simulink model "VSI_fed_Induction_motor"  (R2021a)
settings: Solver=VariableStepAuto  StartTime=0.0  StopTime=10.0  RelTol=1e-3
undefined symbols (not defined in the file): Ts
libraries: spsStairGeneratorLib x3, spsVoltageMeasurementLib x3, spsThreePhaseSourceLib x1, spsMultimeterLib x1, electricdrivelib x1, spspowerguiLib x1
settings Model: Creator=suchi  LastModifiedBy=suchi

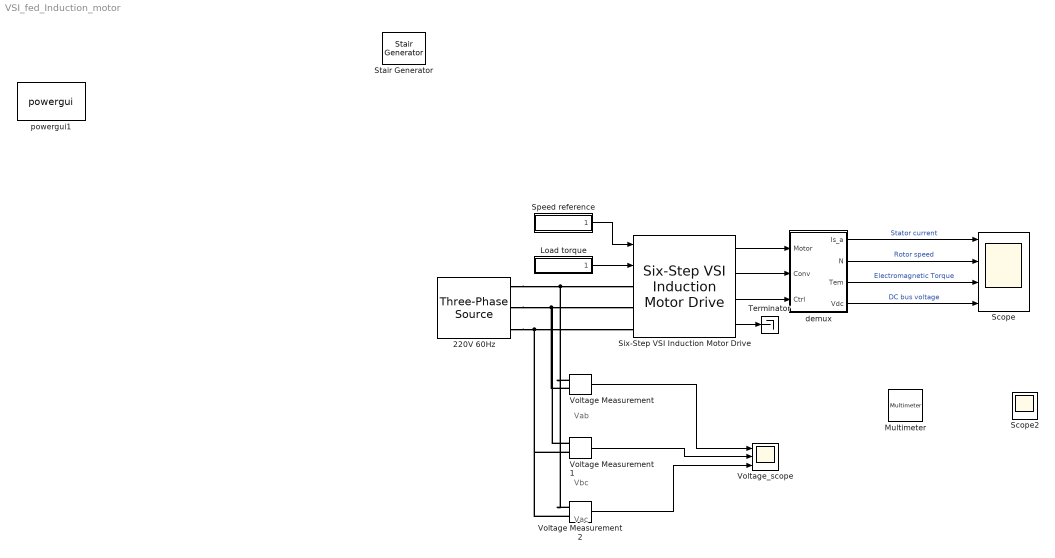
== system VSI_fed_Induction_motor ==
  note: Vac
  note: Vbc
  note: Vab
  220V 60Hz : spsThreePhaseSourceLib/Three-Phase Source  InternalConnection=Yg  VoltagePhases=off  Voltage=220  PhaseAngle=0  Voltage_phases=[25e3 25e3 25e3]/sqrt(3)  PhaseAngles_phases=[0 -120 +120]  Frequency=60  NonIdealSource=on  SpecifyImpedance=off  Resistance=0.1  Inductance=0.1e-3  ShortCircuitLevel=0  BaseVoltage=0  XRratio=0  BusType=swing  Pref=0  Qref=0  Prefabc=[10e3, 10e3, 10e3]  Qrefabc=[0, 0, 0]  Qmin=-inf  Qmax=inf
  Load torque : Subsystem
  Multimeter : spsMultimeterLib/Multimeter  PhasorSimulation=off  OutputType=Complex  sel=1  L=1  Gain=0  yselected={}  PSBOutputType=1  PSBequivalent=0  AxesSetting=[0,0.1,-100,100]  Display=0  SavedBlockNames=-11
  Scope : Scope  NumInputPorts=4
  Scope2 : Scope
  Six-Step VSI Induction Motor Drive : electricdrivelib/AC drives/Six-Step VSI Induction Motor Drive  ReferenceFrame=Stationary  IterativeDiscreteModel=Trapezoidal non iterative  Pn=2238  Vn=220  fn=60  Rs=0.435  Lls=0.002  Lms=69.31e-3  Rr=0.816  Llr=0.002  ia=0  pha=0  ib=0  phb=0  ic=0  phc=0  J=0.089  Friction=0.005  p=2  slip=1  thdeg=0  Rsnb_rec=5e3  Csnb_rec=100e-9  Ron_rec=1e-3  Vf_rec=1.3  ind_bus=1e-3  cap_bus=4000e-6  Rbrake=8  fbrake=4000  deviceType=IGBT / Diodes  Ron_inv=1e-3  Vf_inv=1.7  Vfd_inv=1.7  Tf=1e-6  Tt=2e-6  Tf_GTO=10e-6  Tt_GTO=20e-6  Rsnb_inv=1e3  Csnb_inv=20e-9  fc_busc=30  network_freq=60  bus_dev_neg=20  bus_dev_pos=20  kp_busc=0.01  ki_busc=0.1  busVolt_min=30  busVolt_max=280  Acc=2000  Dec=-2000  outfreq_min=0  outfreq_max=120  vh_ratio=5  zc_time=0.5  baseSampleTime=2e-05  outputBusMode=Multiple output buses  busLabels=off  MechanicalLoad=Torque Tm  driveType=AC1  AverageValue=off
      settings: SourceProductBaseCode=PS
  Speed reference : Subsystem
  Stair Generator : spsStairGeneratorLib/Stair Generator  t=[0, 1, 3, 3.5]  e=[1, -1, 2.5, 0]  Ts=0
  Terminator : Terminator
  Voltage Measurement : spsVoltageMeasurementLib/Voltage Measurement  PhasorSimulation=off  OutputType=Complex  PSBequivalent=0
  Voltage Measurement1 : spsVoltageMeasurementLib/Voltage Measurement  PhasorSimulation=off  OutputType=Complex  PSBequivalent=0
  Voltage Measurement2 : spsVoltageMeasurementLib/Voltage Measurement  PhasorSimulation=off  OutputType=Complex  PSBequivalent=0
  Voltage_scope : Scope  NumInputPorts=3
  demux : Subsystem
  powergui1 : spspowerguiLib/powergui  Priority=2  SimulationMode=Discrete  SampleTime=Ts  frequency=60  Iterations=50  frequencyindice=60  Pbase=100e6  ErrMax=1e-4  UnitsV=kV  UnitsW=MW  buscounter=0  FunctionMessages=off  echomessages=off  EnableUseOfTLC=off  CurrentSourceSwitches=off  DisableSnubberDevices=off  DisableRonSwitches=off  DisableVfSwitches=off  DisplayEquations=off  AutomaticDiscreteSolvers=off  SolverType=Tustin/Backward Euler (TBE)  Interpol=off  ExternalGateDelay=off  methode=off  Ts=0  x0status=blocks  SPID=off  SwTol=0  HookPort=off  NonlinearTolerance=1e-4  nMaxIteration=100  ContinueOnMaxIteration=off  RestoreLinks=warning  ResistiveCurrentMeasurement=off  Frange=[0:2:500]  Ylog=off  Xlog=on  ShowGrid=off  save=off  variable=ZData  structure=0  ZoomFFT=on  StartTime=0.0  cycles=1  DisplayStyle=1  fundamental=60  FreqAxis=off  MaxFrequency=1000  frequencyindicesteady=1  RmsSteady=1  display=off
  wires:
  Six-Step VSI Induction Motor Drive/2 -> demux/2(Conv)
  Load torque/1(" ") -> Six-Step VSI Induction Motor Drive/2
  demux/3(Tem) -> Scope/3  "Electromagnetic Torque"
  demux/4(Vdc) -> Scope/4  "DC bus voltage"
  Six-Step VSI Induction Motor Drive/4 -> Terminator/1
  demux/1(Is_a) -> Scope/1  "Stator current"
  Six-Step VSI Induction Motor Drive/3 -> demux/3(Ctrl)
  Six-Step VSI Induction Motor Drive/1 -> demux/1(Motor)
  demux/2(N) -> Scope/2  "Rotor speed"
  Speed reference/1(" ") -> Six-Step VSI Induction Motor Drive/1
  Voltage Measurement/1 -> Voltage_scope/1
  Voltage Measurement1/1 -> Voltage_scope/2
  Voltage Measurement2/1 -> Voltage_scope/3
  connections:
  220V 60Hz/RConn3 -- Voltage Measurement2/LConn2 -- Voltage Measurement1/LConn2 -- Six-Step VSI Induction Motor Drive/LConn3
  220V 60Hz/RConn1 -- Voltage Measurement2/LConn1 -- Voltage Measurement/LConn1 -- Six-Step VSI Induction Motor Drive/LConn1
  220V 60Hz/RConn2 -- Voltage Measurement1/LConn1 -- Voltage Measurement/LConn2 -- Six-Step VSI Induction Motor Drive/LConn2

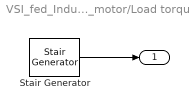
== system VSI_fed_Induction_motor/Load torque ==
  Stair Generator : spsStairGeneratorLib/Stair Generator  t=[ 0 2 3 4]  e=[0 -11 11 0]  Ts=Ts
  " " : Outport  VectorParamsAs1DForOutWhenUnconnected=off
  wires:
  Stair Generator/1 -> " "/1

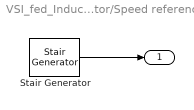
== system VSI_fed_Induction_motor/Speed reference ==
  Stair Generator : spsStairGeneratorLib/Stair Generator  t=[0]  e=[1800]  Ts=Ts
  " " : Outport  VectorParamsAs1DForOutWhenUnconnected=off
  wires:
  Stair Generator/1 -> " "/1

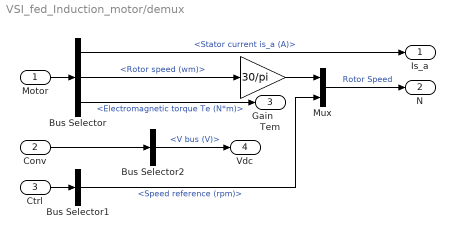
== system VSI_fed_Induction_motor/demux ==
  Motor : Inport
  Conv : Inport  Port=2
  Ctrl : Inport  Port=3
  Bus Selector : BusSelector  OutputSignals=Stator measurements.Stator current is_a (A),Mechanical.Rotor speed (wm),Mechanical.Electromagnetic torque Te (N*m)
  Bus Selector1 : BusSelector  OutputSignals=Speed reference (rpm)
  Bus Selector2 : BusSelector  OutputSignals=V bus (V)
  Gain : Gain  Gain=30/pi  SaturateOnIntegerOverflow=on  OutDataTypeStr=Inherit: Same as input  ParamDataTypeStr=Inherit: Same as input
  Mux : Mux  Inputs=2
  Is_a : Outport  VectorParamsAs1DForOutWhenUnconnected=off
  N : Outport  Port=2  VectorParamsAs1DForOutWhenUnconnected=off
  Tem : Outport  Port=3  VectorParamsAs1DForOutWhenUnconnected=off
  Vdc : Outport  Port=4  VectorParamsAs1DForOutWhenUnconnected=off
  wires:
  Bus Selector/2 -> Gain/1  "<Rotor speed (wm)>"
  Gain/1 -> Mux/1
  Bus Selector1/1 -> Mux/2  "<Speed reference (rpm)>"
  Bus Selector/1 -> Is_a/1  "<Stator current is_a (A)>"
  Motor/1 -> Bus Selector/1
  Mux/1 -> N/1  "Rotor Speed"
  Bus Selector/3 -> Tem/1  "<Electromagnetic torque Te (N*m)>"
  Conv/1 -> Bus Selector2/1
  Ctrl/1 -> Bus Selector1/1
  Bus Selector2/1 -> Vdc/1  "<V bus (V)>"
